simulink model "sampleModel7293_pp_1_1"  (R2018a)
settings: Solver=VariableStepAuto  StartTime=0.0  StopTime=10.0  RelTol=1e-3
undefined symbols (not defined in the file): DiscIntNeverNeededParam
libraries: simulink x367
(part 7 of 12)

== system sampleModel7293_pp_1_1/cfblk175/cfblk17 ==
  cfblk1 : Inport
  cfblk14 : Inport  Port=2
  Action Port : ActionPort  ActionType=else
  cfblk10 : simulink/Continuous/PID Controller (2DOF)  Controller=PID  TimeDomain=Discrete-time  SampleTime=-1  IntegratorMethod=Forward Euler  FilterMethod=Forward Euler  Form=Parallel  UseFilter=on  ControllerParametersSource=internal  P=1  I=1  D=0  N=100  b=1  c=1  InitialConditionSource=internal  InitialConditionForIntegrator=0  InitialConditionForFilter=0  ExternalReset=none  LimitOutput=off  UpperSaturationLimit=inf  LowerSaturationLimit=-inf  LinearizeAsGain=off  AntiWindupMode=none  Kb=1  TrackingMode=off  Kt=1  PParamMin=[]  PParamMax=[]  IParamMin=[]  IParamMax=[]  DParamMin=[]  DParamMax=[]  NParamMin=[]  NParamMax=[]  bParamMin=[]  bParamMax=[]  cParamMin=[]  cParamMax=[]  KbParamMin=[]  KbParamMax=[]  KtParamMin=[]  KtParamMax=[]  POutMin=[]  POutMax=[]  IOutMin=[]  IOutMax=[]  DOutMin=[]  DOutMax=[]  NOutMin=[]  NOutMax=[]  bOutMin=[]  bOutMax=[]  cOutMin=[]  cOutMax=[]  KbOutMin=[]  KbOutMax=[]  KtOutMin=[]  KtOutMax=[]  IntegratorOutMin=[]  IntegratorOutMax=[]  FilterOutMin=[]  FilterOutMax=[]  SumOutMin=[]  SumOutMax=[]  Sum1OutMin=[]  Sum1OutMax=[]  Sum2OutMin=[]  Sum2OutMax=[]  Sum3OutMin=[]  Sum3OutMax=[]  SumI1OutMin=[]  SumI1OutMax=[]  SumI2OutMin=[]  SumI2OutMax=[]  SumI3OutMin=[]  SumI3OutMax=[]  SumDOutMin=[]  SumDOutMax=[]  SaturationOutMin=[]  SaturationOutMax=[]  IntegratorContinuousStateAttributes=''  IntegratorStateMustResolveToSignalObject=off  IntegratorRTWStateStorageClass=Auto  FilterContinuousStateAttributes=''  FilterStateMustResolveToSignalObject=off  FilterRTWStateStorageClass=Auto  DifferentiatorICPrevScaledInput=0  DifferentiatorOutMin=[]  DifferentiatorOutMax=[]  FilterDiffOutCoefMin=[]  FilterDiffOutCoefMax=[]  SumDenOutMin=[]  SumDenOutMax=[]  SumNumOutMin=[]  SumNumOutMax=[]  ReciprocalOutMin=[]  ReciprocalOutMax=[]  DivideOutMin=[]  DivideOutMax=[]  TunerSelectOption=Transfer Function Based (PID Tuner App)
  cfblk11 : simulink/Discrete/Difference  ICPrevInput=0.0  OutMin=[]  OutMax=[]  OutDataTypeStr=double  OutputDataTypeScalingMode=double  OutDataType=fixdt(1, 16)  OutScaling=2^-10  DoSatur=off
  cfblk12 : simulink/Continuous/PID Controller (2DOF)  Controller=PID  TimeDomain=Discrete-time  SampleTime=-1  IntegratorMethod=Forward Euler  FilterMethod=Forward Euler  Form=Parallel  UseFilter=on  ControllerParametersSource=internal  P=1  I=1  D=0  N=100  b=1  c=1  InitialConditionSource=internal  InitialConditionForIntegrator=0  InitialConditionForFilter=0  ExternalReset=none  LimitOutput=off  UpperSaturationLimit=inf  LowerSaturationLimit=-inf  LinearizeAsGain=off  AntiWindupMode=none  Kb=1  TrackingMode=off  Kt=1  PParamMin=[]  PParamMax=[]  IParamMin=[]  IParamMax=[]  DParamMin=[]  DParamMax=[]  NParamMin=[]  NParamMax=[]  bParamMin=[]  bParamMax=[]  cParamMin=[]  cParamMax=[]  KbParamMin=[]  KbParamMax=[]  KtParamMin=[]  KtParamMax=[]  POutMin=[]  POutMax=[]  IOutMin=[]  IOutMax=[]  DOutMin=[]  DOutMax=[]  NOutMin=[]  NOutMax=[]  bOutMin=[]  bOutMax=[]  cOutMin=[]  cOutMax=[]  KbOutMin=[]  KbOutMax=[]  KtOutMin=[]  KtOutMax=[]  IntegratorOutMin=[]  IntegratorOutMax=[]  FilterOutMin=[]  FilterOutMax=[]  SumOutMin=[]  SumOutMax=[]  Sum1OutMin=[]  Sum1OutMax=[]  Sum2OutMin=[]  Sum2OutMax=[]  Sum3OutMin=[]  Sum3OutMax=[]  SumI1OutMin=[]  SumI1OutMax=[]  SumI2OutMin=[]  SumI2OutMax=[]  SumI3OutMin=[]  SumI3OutMax=[]  SumDOutMin=[]  SumDOutMax=[]  SaturationOutMin=[]  SaturationOutMax=[]  IntegratorContinuousStateAttributes=''  IntegratorStateMustResolveToSignalObject=off  IntegratorRTWStateStorageClass=Auto  FilterContinuousStateAttributes=''  FilterStateMustResolveToSignalObject=off  FilterRTWStateStorageClass=Auto  DifferentiatorICPrevScaledInput=0  DifferentiatorOutMin=[]  DifferentiatorOutMax=[]  FilterDiffOutCoefMin=[]  FilterDiffOutCoefMax=[]  SumDenOutMin=[]  SumDenOutMax=[]  SumNumOutMin=[]  SumNumOutMax=[]  ReciprocalOutMin=[]  ReciprocalOutMax=[]  DivideOutMin=[]  DivideOutMax=[]  TunerSelectOption=Transfer Function Based (PID Tuner App)
  cfblk13 : simulink/Discrete/Transfer Fcn Real Zero  ZeroZ=0.75  ICPrevInput=0.0  DoSatur=off
      settings: SourceProductName=Simulink  SourceProductBaseCode=SL
  cfblk16 : Delay
  cfblk3 : Subsystem  TreatAsAtomicUnit=on
  cfblk4 : simulink/Discrete/Tapped Delay  vinit=0.0  samptime=-1  NumDelays=1  DelayOrder=Oldest  includeCurrent=off
  cfblk5 : Subsystem  TreatAsAtomicUnit=on
  cfblk6 : DiscreteIntegrator  SampleTime=-1  OutDataTypeStr=double  ICPrevOutput=DiscIntNeverNeededParam  ICPrevScaledInput=DiscIntNeverNeededParam
  cfblk7 : DiscreteZeroPole  Poles=[0 0.5]  Gain=1  SampleTime=-1
  cfblk8 : Subsystem  TreatAsAtomicUnit=on
  cfblk9 : DiscreteZeroPole  Poles=[0 0.5]  Gain=1  SampleTime=-1
  cyemi_{344..357} (14 alike) : DataTypeConversion  OutDataTypeStr=double
  emi_1488 : Subsystem  TreatAsAtomicUnit=on
  emi_1490 : If  IfExpression=0 <= u1
  emi_1491 : DataTypeConversion  OutDataTypeStr=double
  emi_2063 : Subsystem  TreatAsAtomicUnit=on
  emi_2065 : If  IfExpression=0 <= u1
  emi_2066 : DataTypeConversion  OutDataTypeStr=double
  emi_274 : Subsystem  TreatAsAtomicUnit=on
  emi_276 : If  IfExpression=0 <= u1
  emi_277 : DataTypeConversion  OutDataTypeStr=double
  cfblk2 : Outport
  cfblk15 : Outport  Port=2
  wires:
  cfblk7/1 -> cfblk15/1
  cfblk10/1 -> cfblk2/1
  cfblk12/1 -> cyemi_349/1, cyemi_350/1
  cfblk6/1 -> cyemi_345/1, cyemi_357/1
  cyemi_344/1 -> cfblk10/1
  cfblk13/1 -> cyemi_344/1
  cyemi_345/1 -> cfblk10/2
  cyemi_346/1 -> cfblk11/1
  cfblk9/1 -> cyemi_346/1
  cyemi_347/1 -> cfblk12/1
  cyemi_348/1 -> cfblk12/2
  cfblk14/1 -> cyemi_348/1
  cyemi_349/1 -> cfblk13/1
  cyemi_350/1 -> cfblk16/1
  cyemi_352/1 -> cfblk4/1
  cfblk16/1 -> cyemi_353/1, emi_1491/1, emi_2066/1
  cyemi_354/1 -> cfblk6/1
  cfblk4/1 -> cyemi_354/1, emi_277/1
  cyemi_355/1 -> cfblk7/1
  cfblk11/1 -> cyemi_355/1
  cfblk1/1 -> cyemi_356/1
  cyemi_357/1 -> cfblk9/1
  cyemi_351/1 -> cfblk3/1(emi_272)
  cfblk3/1(emi_273) -> cyemi_352/1
  emi_276/1 -> cfblk3/Action
  emi_276/2 -> emi_274/Action
  emi_277/1 -> emi_276/1
  cyemi_353/1 -> cfblk5/1(emi_1486)
  cfblk5/1(emi_1487) -> cyemi_347/1
  emi_1490/1 -> cfblk5/Action
  emi_1490/2 -> emi_1488/Action
  emi_1491/1 -> emi_1490/1
  cyemi_356/1 -> cfblk8/1(emi_2061)
  cfblk8/1(emi_2062) -> cyemi_351/1
  emi_2065/1 -> cfblk8/Action
  emi_2065/2 -> emi_2063/Action
  emi_2066/1 -> emi_2065/1

== system sampleModel7293_pp_1_1/cfblk175/cfblk5 ==
  emi_193 : Inport
  emi_194 : Inport  Port=2
  Action Port : ActionPort  ActionType=then
  cfblk5 : simulink/Continuous/PID Controller (2DOF)  Controller=PID  TimeDomain=Discrete-time  SampleTime=-1  IntegratorMethod=Forward Euler  FilterMethod=Forward Euler  Form=Parallel  UseFilter=on  ControllerParametersSource=internal  P=1  I=1  D=0  N=100  b=1  c=1  InitialConditionSource=internal  InitialConditionForIntegrator=0  InitialConditionForFilter=0  ExternalReset=none  LimitOutput=off  UpperSaturationLimit=inf  LowerSaturationLimit=-inf  LinearizeAsGain=off  AntiWindupMode=none  Kb=1  TrackingMode=off  Kt=1  PParamMin=[]  PParamMax=[]  IParamMin=[]  IParamMax=[]  DParamMin=[]  DParamMax=[]  NParamMin=[]  NParamMax=[]  bParamMin=[]  bParamMax=[]  cParamMin=[]  cParamMax=[]  KbParamMin=[]  KbParamMax=[]  KtParamMin=[]  KtParamMax=[]  POutMin=[]  POutMax=[]  IOutMin=[]  IOutMax=[]  DOutMin=[]  DOutMax=[]  NOutMin=[]  NOutMax=[]  bOutMin=[]  bOutMax=[]  cOutMin=[]  cOutMax=[]  KbOutMin=[]  KbOutMax=[]  KtOutMin=[]  KtOutMax=[]  IntegratorOutMin=[]  IntegratorOutMax=[]  FilterOutMin=[]  FilterOutMax=[]  SumOutMin=[]  SumOutMax=[]  Sum1OutMin=[]  Sum1OutMax=[]  Sum2OutMin=[]  Sum2OutMax=[]  Sum3OutMin=[]  Sum3OutMax=[]  SumI1OutMin=[]  SumI1OutMax=[]  SumI2OutMin=[]  SumI2OutMax=[]  SumI3OutMin=[]  SumI3OutMax=[]  SumDOutMin=[]  SumDOutMax=[]  SaturationOutMin=[]  SaturationOutMax=[]  IntegratorContinuousStateAttributes=''  IntegratorStateMustResolveToSignalObject=off  IntegratorRTWStateStorageClass=Auto  FilterContinuousStateAttributes=''  FilterStateMustResolveToSignalObject=off  FilterRTWStateStorageClass=Auto  DifferentiatorICPrevScaledInput=0  DifferentiatorOutMin=[]  DifferentiatorOutMax=[]  FilterDiffOutCoefMin=[]  FilterDiffOutCoefMax=[]  SumDenOutMin=[]  SumDenOutMax=[]  SumNumOutMin=[]  SumNumOutMax=[]  ReciprocalOutMin=[]  ReciprocalOutMax=[]  DivideOutMin=[]  DivideOutMax=[]  TunerSelectOption=Transfer Function Based (PID Tuner App)
  emi_195 : Outport
  wires:
  emi_193/1 -> cfblk5/1
  emi_194/1 -> cfblk5/2
  cfblk5/1 -> emi_195/1

== system sampleModel7293_pp_1_1/cfblk175/cfblk6 ==
  emi_502 : Inport
  Action Port : ActionPort  ActionType=then
  cfblk6 : DiscreteFilter
  emi_503 : Outport
  wires:
  emi_502/1 -> cfblk6/1
  cfblk6/1 -> emi_503/1

== system sampleModel7293_pp_1_1/cfblk175/cfblk7 ==
  emi_987 : Inport
  Action Port : ActionPort  ActionType=then
  cfblk7 : DiscreteZeroPole  Poles=[0 0.5]  Gain=1  SampleTime=-1
  emi_988 : Outport
  wires:
  emi_987/1 -> cfblk7/1
  cfblk7/1 -> emi_988/1

== system sampleModel7293_pp_1_1/cfblk175/cfblk8 ==
  emi_315 : Inport
  Action Port : ActionPort  ActionType=then
  cfblk8 : DiscreteFilter
  emi_316 : Outport
  wires:
  emi_315/1 -> cfblk8/1
  cfblk8/1 -> emi_316/1

== system sampleModel7293_pp_1_1/cfblk175/emi_196 ==
  Action Port : ActionPort  ActionType=else
  emi_197 : Assertion

== system sampleModel7293_pp_1_1/cfblk175/emi_317 ==
  Action Port : ActionPort  ActionType=else
  emi_318 : Assertion

== system sampleModel7293_pp_1_1/cfblk175/emi_504 ==
  Action Port : ActionPort  ActionType=else
  emi_505 : Assertion

== system sampleModel7293_pp_1_1/cfblk175/emi_989 ==
  Action Port : ActionPort  ActionType=else
  emi_990 : Assertion

== system sampleModel7293_pp_1_1/cfblk177/cfblk8 ==
  emi_50 : Inport
  Action Port : ActionPort  ActionType=then
  cfblk8 : DiscreteIntegrator  SampleTime=-1  OutDataTypeStr=double  ICPrevOutput=DiscIntNeverNeededParam  ICPrevScaledInput=DiscIntNeverNeededParam
  emi_51 : Outport
  wires:
  emi_50/1 -> cfblk8/1
  cfblk8/1 -> emi_51/1

== system sampleModel7293_pp_1_1/cfblk177/emi_52 ==
  Action Port : ActionPort  ActionType=else
  emi_53 : Assertion

== system sampleModel7293_pp_1_1/cfblk178/cfblk3 ==
  emi_1650 : Inport
  Action Port : ActionPort  ActionType=then
  cfblk3 : simulink/Discrete/Transfer Fcn Real Zero  ZeroZ=0.75  ICPrevInput=0.0  DoSatur=off
      settings: SourceProductName=Simulink  SourceProductBaseCode=SL
  emi_1651 : Outport
  wires:
  emi_1650/1 -> cfblk3/1
  cfblk3/1 -> emi_1651/1

== system sampleModel7293_pp_1_1/cfblk178/cfblk4 ==
  emi_746 : Inport
  Action Port : ActionPort  ActionType=then
  cfblk4 : DiscreteIntegrator  SampleTime=-1  OutDataTypeStr=double  ICPrevOutput=DiscIntNeverNeededParam  ICPrevScaledInput=DiscIntNeverNeededParam
  emi_747 : Outport
  wires:
  emi_746/1 -> cfblk4/1
  cfblk4/1 -> emi_747/1

== system sampleModel7293_pp_1_1/cfblk178/cfblk9 ==
  emi_2019 : Inport
  Action Port : ActionPort  ActionType=then
  cfblk9 : DiscreteZeroPole  Poles=[0 0.5]  Gain=1  SampleTime=-1
  emi_2020 : Outport
  wires:
  emi_2019/1 -> cfblk9/1
  cfblk9/1 -> emi_2020/1

== system sampleModel7293_pp_1_1/cfblk178/emi_1652 ==
  Action Port : ActionPort  ActionType=else
  emi_1653 : Assertion

== system sampleModel7293_pp_1_1/cfblk178/emi_2021 ==
  Action Port : ActionPort  ActionType=else
  emi_2022 : Assertion

== system sampleModel7293_pp_1_1/cfblk178/emi_748 ==
  Action Port : ActionPort  ActionType=else
  emi_749 : Assertion

== system sampleModel7293_pp_1_1/cfblk179/cfblk16 ==
  emi_1287 : Inport
  Action Port : ActionPort  ActionType=then
  cfblk16 : Delay
  emi_1288 : Outport
  wires:
  emi_1287/1 -> cfblk16/1
  cfblk16/1 -> emi_1288/1

== system sampleModel7293_pp_1_1/cfblk179/cfblk7 ==
  emi_57 : Inport
  Action Port : ActionPort  ActionType=then
  cfblk7 : simulink/Discrete/Transfer Fcn Lead or Lag  PoleZ=0.95  ZeroZ=0.75  ICPrevOutput=0.0  ICPrevInput=0.0  DoSatur=off
      settings: SourceProductName=Simulink  SourceProductBaseCode=SL
  emi_58 : Outport
  wires:
  emi_57/1 -> cfblk7/1
  cfblk7/1 -> emi_58/1

== system sampleModel7293_pp_1_1/cfblk179/cfblk8 ==
  emi_1600 : Inport
  Action Port : ActionPort  ActionType=then
  cfblk8 : simulink/Discrete/Transfer Fcn Real Zero  ZeroZ=0.75  ICPrevInput=0.0  DoSatur=off
      settings: SourceProductName=Simulink  SourceProductBaseCode=SL
  emi_1601 : Outport
  wires:
  emi_1600/1 -> cfblk8/1
  cfblk8/1 -> emi_1601/1

== system sampleModel7293_pp_1_1/cfblk179/emi_1289 ==
  Action Port : ActionPort  ActionType=else
  emi_1290 : Assertion

== system sampleModel7293_pp_1_1/cfblk179/emi_1602 ==
  Action Port : ActionPort  ActionType=else
  emi_1603 : Assertion

== system sampleModel7293_pp_1_1/cfblk179/emi_59 ==
  Action Port : ActionPort  ActionType=else
  emi_60 : Assertion

== system sampleModel7293_pp_1_1/cfblk180/cfblk17 ==
  cfblk1 : Inport
  Action Port : ActionPort  ActionType=then
  cfblk10 : Delay
  cfblk3 : Subsystem  TreatAsAtomicUnit=on
  cfblk4 : Delay  ShowEnablePort=on
      settings: InputPortMap=u0,e6
  cfblk5 : Subsystem  TreatAsAtomicUnit=on
  cfblk6 : DiscreteTransferFcn
  cfblk7 : Subsystem  TreatAsAtomicUnit=on
  cfblk8 : Subsystem  TreatAsAtomicUnit=on
  cfblk9 : Subsystem  TreatAsAtomicUnit=on
  cyemi_{429..439} (11 alike) : DataTypeConversion  OutDataTypeStr=double
  emi_110 : Subsystem  TreatAsAtomicUnit=on
  emi_{112,356,822,1505,1931} (5 alike) : If  IfExpression=Inf <= u1
  emi_{113,357,823,1506,1932} (5 alike) : DataTypeConversion  OutDataTypeStr=double
  emi_1503 : Subsystem  TreatAsAtomicUnit=on
  emi_1929 : Subsystem  TreatAsAtomicUnit=on
  emi_354 : Subsystem  TreatAsAtomicUnit=on
  emi_820 : Subsystem  TreatAsAtomicUnit=on
  cfblk2 : Outport
  wires:
  cfblk1/1 -> cyemi_434/1, cyemi_436/1, cyemi_437/1
  cyemi_429/1 -> cfblk10/1
  cfblk6/1 -> cyemi_431/1, emi_823/1
  cyemi_432/1 -> cfblk4/1
  cyemi_433/1 -> cfblk4/2
  cfblk10/1 -> cyemi_433/1, emi_1506/1, emi_1932/1
  cyemi_435/1 -> cfblk6/1
  cfblk4/1 -> cyemi_439/1, emi_357/1
  cyemi_439/1 -> cfblk9/1(emi_108)
  cfblk9/1(emi_109) -> cyemi_438/1, cyemi_430/1
  emi_112/1 -> cfblk9/Action
  emi_112/2 -> emi_110/Action
  emi_113/1 -> emi_112/1
  cyemi_438/1 -> cfblk8/1(emi_352)
  cfblk8/1(emi_353) -> cyemi_429/1
  emi_356/1 -> cfblk8/Action
  emi_356/2 -> emi_354/Action
  emi_357/1 -> emi_356/1
  cyemi_430/1 -> cfblk3/1(emi_817)
  cyemi_431/1 -> cfblk3/2(emi_818)
  cfblk3/1(emi_819) -> cfblk2/1
  emi_822/1 -> cfblk3/Action
  emi_822/2 -> emi_820/Action
  emi_823/1 -> emi_822/1
  cyemi_436/1 -> cfblk7/1(emi_1500)
  cyemi_437/1 -> cfblk7/2(emi_1501)
  cfblk7/1(emi_1502) -> cyemi_435/1
  emi_1505/1 -> cfblk7/Action
  emi_1505/2 -> emi_1503/Action
  emi_1506/1 -> emi_1505/1
  cyemi_434/1 -> cfblk5/1(emi_1927)
  cfblk5/1(emi_1928) -> emi_113/1, cyemi_432/1
  emi_1931/1 -> cfblk5/Action
  emi_1931/2 -> emi_1929/Action
  emi_1932/1 -> emi_1931/1

== system sampleModel7293_pp_1_1/cfblk180/cfblk18 ==
  cfblk1 : Inport
  Action Port : ActionPort  ActionType=else
  cfblk10 : Subsystem  TreatAsAtomicUnit=on
  cfblk11 : simulink/Continuous/PID Controller  Controller=PID  TimeDomain=Discrete-time  SampleTime=-1  IntegratorMethod=Forward Euler  FilterMethod=Forward Euler  Form=Parallel  UseFilter=on  ControllerParametersSource=internal  P=1  I=1  D=0  N=100  InitialConditionSource=internal  InitialConditionForIntegrator=0  InitialConditionForFilter=0  ExternalReset=none  LimitOutput=off  UpperSaturationLimit=inf  LowerSaturationLimit=-inf  LinearizeAsGain=off  AntiWindupMode=none  Kb=1  TrackingMode=off  Kt=1  PParamMin=[]  PParamMax=[]  IParamMin=[]  IParamMax=[]  DParamMin=[]  DParamMax=[]  NParamMin=[]  NParamMax=[]  KbParamMin=[]  KbParamMax=[]  KtParamMin=[]  KtParamMax=[]  POutMin=[]  POutMax=[]  IOutMin=[]  IOutMax=[]  DOutMin=[]  DOutMax=[]  NOutMin=[]  NOutMax=[]  KbOutMin=[]  KbOutMax=[]  KtOutMin=[]  KtOutMax=[]  IntegratorOutMin=[]  IntegratorOutMax=[]  FilterOutMin=[]  FilterOutMax=[]  SumOutMin=[]  SumOutMax=[]  SumI1OutMin=[]  SumI1OutMax=[]  SumI2OutMin=[]  SumI2OutMax=[]  SumI3OutMin=[]  SumI3OutMax=[]  SumDOutMin=[]  SumDOutMax=[]  SaturationOutMin=[]  SaturationOutMax=[]  IntegratorContinuousStateAttributes=''  IntegratorStateMustResolveToSignalObject=off  IntegratorRTWStateStorageClass=Auto  FilterContinuousStateAttributes=''  FilterStateMustResolveToSignalObject=off  FilterRTWStateStorageClass=Auto  DifferentiatorICPrevScaledInput=0  DifferentiatorOutMin=[]  DifferentiatorOutMax=[]  FilterDiffOutCoefMin=[]  FilterDiffOutCoefMax=[]  SumDenOutMin=[]  SumDenOutMax=[]  SumNumOutMin=[]  SumNumOutMax=[]  ReciprocalOutMin=[]  ReciprocalOutMax=[]  DivideOutMin=[]  DivideOutMax=[]  TunerSelectOption=Transfer Function Based (PID Tuner App)
  cfblk14 : Delay
  cfblk15 : Delay
  cfblk3 : simulink/Discrete/Difference  ICPrevInput=0.0  OutMin=[]  OutMax=[]  OutDataTypeStr=double  OutputDataTypeScalingMode=double  OutDataType=fixdt(1, 16)  OutScaling=2^-10  DoSatur=off
  cfblk4 : simulink/Continuous/PID Controller  Controller=PID  TimeDomain=Discrete-time  SampleTime=-1  IntegratorMethod=Forward Euler  FilterMethod=Forward Euler  Form=Parallel  UseFilter=on  ControllerParametersSource=internal  P=1  I=1  D=0  N=100  InitialConditionSource=internal  InitialConditionForIntegrator=0  InitialConditionForFilter=0  ExternalReset=none  LimitOutput=off  UpperSaturationLimit=inf  LowerSaturationLimit=-inf  LinearizeAsGain=off  AntiWindupMode=none  Kb=1  TrackingMode=off  Kt=1  PParamMin=[]  PParamMax=[]  IParamMin=[]  IParamMax=[]  DParamMin=[]  DParamMax=[]  NParamMin=[]  NParamMax=[]  KbParamMin=[]  KbParamMax=[]  KtParamMin=[]  KtParamMax=[]  POutMin=[]  POutMax=[]  IOutMin=[]  IOutMax=[]  DOutMin=[]  DOutMax=[]  NOutMin=[]  NOutMax=[]  KbOutMin=[]  KbOutMax=[]  KtOutMin=[]  KtOutMax=[]  IntegratorOutMin=[]  IntegratorOutMax=[]  FilterOutMin=[]  FilterOutMax=[]  SumOutMin=[]  SumOutMax=[]  SumI1OutMin=[]  SumI1OutMax=[]  SumI2OutMin=[]  SumI2OutMax=[]  SumI3OutMin=[]  SumI3OutMax=[]  SumDOutMin=[]  SumDOutMax=[]  SaturationOutMin=[]  SaturationOutMax=[]  IntegratorContinuousStateAttributes=''  IntegratorStateMustResolveToSignalObject=off  IntegratorRTWStateStorageClass=Auto  FilterContinuousStateAttributes=''  FilterStateMustResolveToSignalObject=off  FilterRTWStateStorageClass=Auto  DifferentiatorICPrevScaledInput=0  DifferentiatorOutMin=[]  DifferentiatorOutMax=[]  FilterDiffOutCoefMin=[]  FilterDiffOutCoefMax=[]  SumDenOutMin=[]  SumDenOutMax=[]  SumNumOutMin=[]  SumNumOutMax=[]  ReciprocalOutMin=[]  ReciprocalOutMax=[]  DivideOutMin=[]  DivideOutMax=[]  TunerSelectOption=Transfer Function Based (PID Tuner App)
  cfblk5 : Subsystem  TreatAsAtomicUnit=on
  cfblk6 : Delay
  cfblk7 : Subsystem  TreatAsAtomicUnit=on
  cfblk8 : Delay  DelayLengthSource=Input port
      settings: InputPortMap=u0,p1
  cfblk9 : Delay  ShowEnablePort=on
      settings: InputPortMap=u0,e6
  cyemi_{441..454} (14 alike) : DataTypeConversion  OutDataTypeStr=double
  emi_2085 : Subsystem  TreatAsAtomicUnit=on
  emi_2087 : If  IfExpression=Inf <= u1
  emi_2088 : DataTypeConversion  OutDataTypeStr=double
  emi_2107 : Subsystem  TreatAsAtomicUnit=on
  emi_2109 : If  IfExpression=Inf <= u1
  emi_2110 : DataTypeConversion  OutDataTypeStr=double
  emi_238 : Subsystem  TreatAsAtomicUnit=on
  emi_240 : If  IfExpression=Inf <= u1
  emi_241 : DataTypeConversion  OutDataTypeStr=double
  cfblk2 : Outport
  cfblk12 : Outport  Port=2
  cfblk13 : Outport  Port=3
  wires:
  cfblk4/1 -> cyemi_449/1, cyemi_454/1
  cfblk8/1 -> cfblk2/1, cyemi_446/1
  cfblk3/1 -> cyemi_441/1, cyemi_450/1
  cfblk6/1 -> cyemi_445/1, cyemi_453/1, emi_241/1, emi_2088/1
  cyemi_442/1 -> cfblk11/1
  cyemi_443/1 -> cfblk14/1
  cfblk11/1 -> cyemi_443/1
  cyemi_444/1 -> cfblk15/1
  cfblk9/1 -> cyemi_444/1
  cyemi_445/1 -> cfblk3/1
  cyemi_446/1 -> cfblk4/1
  cfblk15/1 -> cyemi_447/1, emi_2110/1
  cfblk1/1 -> cyemi_448/1
  cyemi_449/1 -> cfblk6/1
  cyemi_451/1 -> cfblk8/1
  cyemi_452/1 -> cfblk8/2
  cfblk14/1 -> cyemi_452/1
  cyemi_453/1 -> cfblk9/1
  cyemi_454/1 -> cfblk9/2
  cyemi_450/1 -> cfblk7/1(emi_236)
  cfblk7/1(emi_237) -> cfblk12/1
  emi_240/1 -> cfblk7/Action
  emi_240/2 -> emi_238/Action
  emi_241/1 -> emi_240/1
  cyemi_447/1 -> cfblk5/1(emi_2082)
  cyemi_448/1 -> cfblk5/2(emi_2083)
  cfblk5/1(emi_2084) -> cyemi_451/1, cfblk13/1
  emi_2087/1 -> cfblk5/Action
  emi_2087/2 -> emi_2085/Action
  emi_2088/1 -> emi_2087/1
  cyemi_441/1 -> cfblk10/1(emi_2105)
  cfblk10/1(emi_2106) -> cyemi_442/1
  emi_2109/1 -> cfblk10/Action
  emi_2109/2 -> emi_2107/Action
  emi_2110/1 -> emi_2109/1

== system sampleModel7293_pp_1_1/cfblk180/cfblk4 ==
  emi_1998 : Inport
  Action Port : ActionPort  ActionType=then
  cfblk4 : Delay
  emi_1999 : Outport
  wires:
  emi_1998/1 -> cfblk4/1
  cfblk4/1 -> emi_1999/1

== system sampleModel7293_pp_1_1/cfblk180/cfblk9 ==
  emi_2133 : Inport
  Action Port : ActionPort  ActionType=then
  cfblk9 : DiscreteZeroPole  Poles=[0 0.5]  Gain=1  SampleTime=-1
  emi_2134 : Outport
  wires:
  emi_2133/1 -> cfblk9/1
  cfblk9/1 -> emi_2134/1

== system sampleModel7293_pp_1_1/cfblk180/emi_2000 ==
  Action Port : ActionPort  ActionType=else
  emi_2001 : Assertion

== system sampleModel7293_pp_1_1/cfblk180/emi_2135 ==
  Action Port : ActionPort  ActionType=else
  emi_2136 : Assertion

== system sampleModel7293_pp_1_1/cfblk181/cfblk10 ==
  emi_79 : Inport
  Action Port : ActionPort  ActionType=then
  cfblk10 : Delay
  emi_80 : Outport
  wires:
  emi_79/1 -> cfblk10/1
  cfblk10/1 -> emi_80/1

== system sampleModel7293_pp_1_1/cfblk181/emi_81 ==
  Action Port : ActionPort  ActionType=else
  emi_82 : Assertion

== system sampleModel7293_pp_1_1/cfblk182/cfblk12 ==
  cfblk1 : Inport
  cfblk13 : Inport  Port=2
  cfblk14 : Inport  Port=3
  Action Port : ActionPort  ActionType=then
  cfblk10 : simulink/Discrete/Transfer Fcn Real Zero  ZeroZ=0.75  ICPrevInput=0.0  DoSatur=off
      settings: SourceProductName=Simulink  SourceProductBaseCode=SL
  cfblk11 : simulink/Discrete/Transfer Fcn First Order  PoleZ=0.95  ICPrevOutput=0.0  DoSatur=off
      settings: SourceProductName=Simulink
  cfblk12 : simulink/Discrete/Tapped Delay  vinit=0.0  samptime=-1  NumDelays=1  DelayOrder=Oldest  includeCurrent=off
  cfblk3 : Subsystem  TreatAsAtomicUnit=on
  cfblk4 : DiscreteFir
  cfblk5 : DiscreteFilter
  cfblk6 : DiscreteFir
  cfblk7 : Subsystem  TreatAsAtomicUnit=on
  cfblk8 : Delay  ShowEnablePort=on
      settings: InputPortMap=u0,e6
  cfblk9 : simulink/Continuous/PID Controller  Controller=PID  TimeDomain=Discrete-time  SampleTime=-1  IntegratorMethod=Forward Euler  FilterMethod=Forward Euler  Form=Parallel  UseFilter=on  ControllerParametersSource=internal  P=1  I=1  D=0  N=100  InitialConditionSource=internal  InitialConditionForIntegrator=0  InitialConditionForFilter=0  ExternalReset=none  LimitOutput=off  UpperSaturationLimit=inf  LowerSaturationLimit=-inf  LinearizeAsGain=off  AntiWindupMode=none  Kb=1  TrackingMode=off  Kt=1  PParamMin=[]  PParamMax=[]  IParamMin=[]  IParamMax=[]  DParamMin=[]  DParamMax=[]  NParamMin=[]  NParamMax=[]  KbParamMin=[]  KbParamMax=[]  KtParamMin=[]  KtParamMax=[]  POutMin=[]  POutMax=[]  IOutMin=[]  IOutMax=[]  DOutMin=[]  DOutMax=[]  NOutMin=[]  NOutMax=[]  KbOutMin=[]  KbOutMax=[]  KtOutMin=[]  KtOutMax=[]  IntegratorOutMin=[]  IntegratorOutMax=[]  FilterOutMin=[]  FilterOutMax=[]  SumOutMin=[]  SumOutMax=[]  SumI1OutMin=[]  SumI1OutMax=[]  SumI2OutMin=[]  SumI2OutMax=[]  SumI3OutMin=[]  SumI3OutMax=[]  SumDOutMin=[]  SumDOutMax=[]  SaturationOutMin=[]  SaturationOutMax=[]  IntegratorContinuousStateAttributes=''  IntegratorStateMustResolveToSignalObject=off  IntegratorRTWStateStorageClass=Auto  FilterContinuousStateAttributes=''  FilterStateMustResolveToSignalObject=off  FilterRTWStateStorageClass=Auto  DifferentiatorICPrevScaledInput=0  DifferentiatorOutMin=[]  DifferentiatorOutMax=[]  FilterDiffOutCoefMin=[]  FilterDiffOutCoefMax=[]  SumDenOutMin=[]  SumDenOutMax=[]  SumNumOutMin=[]  SumNumOutMax=[]  ReciprocalOutMin=[]  ReciprocalOutMax=[]  DivideOutMin=[]  DivideOutMax=[]  TunerSelectOption=Transfer Function Based (PID Tuner App)
  cyemi_{480..490} (11 alike) : DataTypeConversion  OutDataTypeStr=double
  emi_103 : Subsystem  TreatAsAtomicUnit=on
  emi_105 : If  IfExpression=Inf <= u1
  emi_106 : DataTypeConversion  OutDataTypeStr=double
  emi_982 : Subsystem  TreatAsAtomicUnit=on
  emi_984 : If  IfExpression=Inf <= u1
  emi_985 : DataTypeConversion  OutDataTypeStr=double
  cfblk2 : Outport
  wires:
  cfblk11/1 -> cfblk2/1
  cyemi_480/1 -> cfblk10/1
  cyemi_481/1 -> cfblk11/1
  cfblk14/1 -> cyemi_481/1
  cyemi_482/1 -> cfblk12/1
  cfblk1/1 -> cyemi_482/1
  cfblk13/1 -> cyemi_483/1
  cyemi_484/1 -> cfblk4/1
  cfblk9/1 -> cyemi_484/1
  cyemi_485/1 -> cfblk5/1
  cfblk4/1 -> cyemi_485/1, emi_106/1
  cyemi_486/1 -> cfblk6/1
  cfblk8/1 -> cyemi_486/1
  cyemi_488/1 -> cfblk8/1
  cfblk12/1 -> cyemi_488/1, emi_985/1
  cyemi_489/1 -> cfblk8/2
  cfblk5/1 -> cyemi_489/1
  cyemi_490/1 -> cfblk9/1
  cfblk10/1 -> cyemi_490/1
  cyemi_487/1 -> cfblk7/1(emi_101)
  cfblk7/1(emi_102) -> cyemi_480/1
  emi_105/1 -> cfblk7/Action
  emi_105/2 -> emi_103/Action
  emi_106/1 -> emi_105/1
  cyemi_483/1 -> cfblk3/1(emi_980)
  cfblk3/1(emi_981) -> cyemi_487/1
  emi_984/1 -> cfblk3/Action
  emi_984/2 -> emi_982/Action
  emi_985/1 -> emi_984/1

== system sampleModel7293_pp_1_1/cfblk182/cfblk13 ==
  cfblk1 : Inport
  cfblk9 : Inport  Port=2
  cfblk10 : Inport  Port=3
  Action Port : ActionPort  ActionType=else
  cfblk11 : Subsystem  TreatAsAtomicUnit=on
  cfblk3 : Subsystem  TreatAsAtomicUnit=on
  cfblk4 : DiscreteIntegrator  SampleTime=-1  OutDataTypeStr=double  ICPrevOutput=DiscIntNeverNeededParam  ICPrevScaledInput=DiscIntNeverNeededParam
  cfblk5 : DiscreteZeroPole  Poles=[0 0.5]  Gain=1  SampleTime=-1
  cfblk6 : DiscreteIntegrator  SampleTime=-1  OutDataTypeStr=double  ICPrevOutput=DiscIntNeverNeededParam  ICPrevScaledInput=DiscIntNeverNeededParam
  cfblk7 : DiscreteZeroPole  Poles=[0 0.5]  Gain=1  SampleTime=-1
  cfblk8 : simulink/Continuous/PID Controller (2DOF)  Controller=PID  TimeDomain=Discrete-time  SampleTime=-1  IntegratorMethod=Forward Euler  FilterMethod=Forward Euler  Form=Parallel  UseFilter=on  ControllerParametersSource=internal  P=1  I=1  D=0  N=100  b=1  c=1  InitialConditionSource=internal  InitialConditionForIntegrator=0  InitialConditionForFilter=0  ExternalReset=none  LimitOutput=off  UpperSaturationLimit=inf  LowerSaturationLimit=-inf  LinearizeAsGain=off  AntiWindupMode=none  Kb=1  TrackingMode=off  Kt=1  PParamMin=[]  PParamMax=[]  IParamMin=[]  IParamMax=[]  DParamMin=[]  DParamMax=[]  NParamMin=[]  NParamMax=[]  bParamMin=[]  bParamMax=[]  cParamMin=[]  cParamMax=[]  KbParamMin=[]  KbParamMax=[]  KtParamMin=[]  KtParamMax=[]  POutMin=[]  POutMax=[]  IOutMin=[]  IOutMax=[]  DOutMin=[]  DOutMax=[]  NOutMin=[]  NOutMax=[]  bOutMin=[]  bOutMax=[]  cOutMin=[]  cOutMax=[]  KbOutMin=[]  KbOutMax=[]  KtOutMin=[]  KtOutMax=[]  IntegratorOutMin=[]  IntegratorOutMax=[]  FilterOutMin=[]  FilterOutMax=[]  SumOutMin=[]  SumOutMax=[]  Sum1OutMin=[]  Sum1OutMax=[]  Sum2OutMin=[]  Sum2OutMax=[]  Sum3OutMin=[]  Sum3OutMax=[]  SumI1OutMin=[]  SumI1OutMax=[]  SumI2OutMin=[]  SumI2OutMax=[]  SumI3OutMin=[]  SumI3OutMax=[]  SumDOutMin=[]  SumDOutMax=[]  SaturationOutMin=[]  SaturationOutMax=[]  IntegratorContinuousStateAttributes=''  IntegratorStateMustResolveToSignalObject=off  IntegratorRTWStateStorageClass=Auto  FilterContinuousStateAttributes=''  FilterStateMustResolveToSignalObject=off  FilterRTWStateStorageClass=Auto  DifferentiatorICPrevScaledInput=0  DifferentiatorOutMin=[]  DifferentiatorOutMax=[]  FilterDiffOutCoefMin=[]  FilterDiffOutCoefMax=[]  SumDenOutMin=[]  SumDenOutMax=[]  SumNumOutMin=[]  SumNumOutMax=[]  ReciprocalOutMin=[]  ReciprocalOutMax=[]  DivideOutMin=[]  DivideOutMax=[]  TunerSelectOption=Transfer Function Based (PID Tuner App)
  cyemi_{494..501} (8 alike) : DataTypeConversion  OutDataTypeStr=double
  emi_1466 : Subsystem  TreatAsAtomicUnit=on
  emi_1468 : If  IfExpression=Inf <= u1
  emi_1469 : DataTypeConversion  OutDataTypeStr=double
  emi_1674 : Subsystem  TreatAsAtomicUnit=on
  emi_1676 : If  IfExpression=Inf <= u1
  emi_1677 : DataTypeConversion  OutDataTypeStr=double
  cfblk2 : Outport
  wires:
  cfblk8/1 -> cyemi_494/1
  cfblk5/1 -> cyemi_495/1, emi_1469/1, emi_1677/1
  cyemi_496/1 -> cfblk4/1
  cfblk1/1 -> cyemi_496/1
  cyemi_497/1 -> cfblk5/1
  cfblk6/1 -> cyemi_497/1
  cyemi_498/1 -> cfblk6/1
  cfblk9/1 -> cyemi_498/1
  cyemi_499/1 -> cfblk7/1
  cyemi_500/1 -> cfblk8/1
  cfblk7/1 -> cyemi_500/1
  cyemi_501/1 -> cfblk8/2
  cfblk10/1 -> cyemi_501/1
  cyemi_494/1 -> cfblk11/1(emi_1464)
  cfblk11/1(emi_1465) -> cyemi_499/1
  emi_1468/1 -> cfblk11/Action
  emi_1468/2 -> emi_1466/Action
  emi_1469/1 -> emi_1468/1
  cyemi_495/1 -> cfblk3/1(emi_1672)
  cfblk3/1(emi_1673) -> cfblk2/1
  emi_1676/1 -> cfblk3/Action
  emi_1676/2 -> emi_1674/Action
  emi_1677/1 -> emi_1676/1

== system sampleModel7293_pp_1_1/cfblk182/cfblk15 ==
  emi_1721 : Inport
  Action Port : ActionPort  ActionType=then
  cfblk15 : Delay
  emi_1722 : Outport
  wires:
  emi_1721/1 -> cfblk15/1
  cfblk15/1 -> emi_1722/1

== system sampleModel7293_pp_1_1/cfblk182/cfblk16 ==
  emi_1422 : Inport
  Action Port : ActionPort  ActionType=then
  cfblk16 : Delay
  emi_1423 : Outport
  wires:
  emi_1422/1 -> cfblk16/1
  cfblk16/1 -> emi_1423/1

== system sampleModel7293_pp_1_1/cfblk182/cfblk3 ==
  emi_603 : Inport
  Action Port : ActionPort  ActionType=then
  cfblk3 : simulink/Discrete/Transfer Fcn Lead or Lag  PoleZ=0.95  ZeroZ=0.75  ICPrevOutput=0.0  ICPrevInput=0.0  DoSatur=off
      settings: SourceProductName=Simulink  SourceProductBaseCode=SL
  emi_604 : Outport
  wires:
  emi_603/1 -> cfblk3/1
  cfblk3/1 -> emi_604/1

== system sampleModel7293_pp_1_1/cfblk182/cfblk6 ==
  emi_896 : Inport
  Action Port : ActionPort  ActionType=then
  cfblk6 : UnitDelay  SampleTime=-1
  emi_897 : Outport
  wires:
  emi_896/1 -> cfblk6/1
  cfblk6/1 -> emi_897/1

== system sampleModel7293_pp_1_1/cfblk182/cfblk9 ==
  emi_1771 : Inport
  emi_1772 : Inport  Port=2
  Action Port : ActionPort  ActionType=then
  cfblk9 : Delay  DelayLengthSource=Input port
      settings: InputPortMap=u0,p1
  emi_1773 : Outport
  wires:
  emi_1771/1 -> cfblk9/1
  emi_1772/1 -> cfblk9/2
  cfblk9/1 -> emi_1773/1

== system sampleModel7293_pp_1_1/cfblk182/emi_1424 ==
  Action Port : ActionPort  ActionType=else
  emi_1425 : Assertion

== system sampleModel7293_pp_1_1/cfblk182/emi_1723 ==
  Action Port : ActionPort  ActionType=else
  emi_1724 : Assertion

== system sampleModel7293_pp_1_1/cfblk182/emi_1774 ==
  Action Port : ActionPort  ActionType=else
  emi_1775 : Assertion

== system sampleModel7293_pp_1_1/cfblk182/emi_605 ==
  Action Port : ActionPort  ActionType=else
  emi_606 : Assertion

== system sampleModel7293_pp_1_1/cfblk182/emi_898 ==
  Action Port : ActionPort  ActionType=else
  emi_899 : Assertion

== system sampleModel7293_pp_1_1/cfblk183/cfblk15 ==
  emi_1850 : Inport
  Action Port : ActionPort  ActionType=then
  cfblk15 : Delay
  emi_1851 : Outport
  wires:
  emi_1850/1 -> cfblk15/1
  cfblk15/1 -> emi_1851/1

== system sampleModel7293_pp_1_1/cfblk183/cfblk3 ==
  emi_1400 : Inport
  emi_1401 : Inport  Port=2
  Action Port : ActionPort  ActionType=then
  cfblk3 : Delay  ShowEnablePort=on
      settings: InputPortMap=u0,e6
  emi_1402 : Outport
  wires:
  emi_1400/1 -> cfblk3/1
  emi_1401/1 -> cfblk3/2
  cfblk3/1 -> emi_1402/1

== system sampleModel7293_pp_1_1/cfblk183/cfblk4 ==
  emi_394 : Inport
  Action Port : ActionPort  ActionType=then
  cfblk4 : DiscreteFilter
  emi_395 : Outport
  wires:
  emi_394/1 -> cfblk4/1
  cfblk4/1 -> emi_395/1

== system sampleModel7293_pp_1_1/cfblk183/cfblk5 ==
  emi_1962 : Inport
  Action Port : ActionPort  ActionType=then
  cfblk5 : DiscreteStateSpace  SampleTime=-1
  emi_1963 : Outport
  wires:
  emi_1962/1 -> cfblk5/1
  cfblk5/1 -> emi_1963/1

== system sampleModel7293_pp_1_1/cfblk183/emi_1403 ==
  Action Port : ActionPort  ActionType=else
  emi_1404 : Assertion

== system sampleModel7293_pp_1_1/cfblk183/emi_1852 ==
  Action Port : ActionPort  ActionType=else
  emi_1853 : Assertion

== system sampleModel7293_pp_1_1/cfblk183/emi_1964 ==
  Action Port : ActionPort  ActionType=else
  emi_1965 : Assertion

== system sampleModel7293_pp_1_1/cfblk183/emi_396 ==
  Action Port : ActionPort  ActionType=else
  emi_397 : Assertion

== system sampleModel7293_pp_1_1/cfblk184/cfblk12 ==
  emi_853 : Inport
  emi_854 : Inport  Port=2
  Action Port : ActionPort  ActionType=then
  cfblk12 : simulink/Continuous/PID Controller (2DOF)  Controller=PID  TimeDomain=Discrete-time  SampleTime=-1  IntegratorMethod=Forward Euler  FilterMethod=Forward Euler  Form=Parallel  UseFilter=on  ControllerParametersSource=internal  P=1  I=1  D=0  N=100  b=1  c=1  InitialConditionSource=internal  InitialConditionForIntegrator=0  InitialConditionForFilter=0  ExternalReset=none  LimitOutput=off  UpperSaturationLimit=inf  LowerSaturationLimit=-inf  LinearizeAsGain=off  AntiWindupMode=none  Kb=1  TrackingMode=off  Kt=1  PParamMin=[]  PParamMax=[]  IParamMin=[]  IParamMax=[]  DParamMin=[]  DParamMax=[]  NParamMin=[]  NParamMax=[]  bParamMin=[]  bParamMax=[]  cParamMin=[]  cParamMax=[]  KbParamMin=[]  KbParamMax=[]  KtParamMin=[]  KtParamMax=[]  POutMin=[]  POutMax=[]  IOutMin=[]  IOutMax=[]  DOutMin=[]  DOutMax=[]  NOutMin=[]  NOutMax=[]  bOutMin=[]  bOutMax=[]  cOutMin=[]  cOutMax=[]  KbOutMin=[]  KbOutMax=[]  KtOutMin=[]  KtOutMax=[]  IntegratorOutMin=[]  IntegratorOutMax=[]  FilterOutMin=[]  FilterOutMax=[]  SumOutMin=[]  SumOutMax=[]  Sum1OutMin=[]  Sum1OutMax=[]  Sum2OutMin=[]  Sum2OutMax=[]  Sum3OutMin=[]  Sum3OutMax=[]  SumI1OutMin=[]  SumI1OutMax=[]  SumI2OutMin=[]  SumI2OutMax=[]  SumI3OutMin=[]  SumI3OutMax=[]  SumDOutMin=[]  SumDOutMax=[]  SaturationOutMin=[]  SaturationOutMax=[]  IntegratorContinuousStateAttributes=''  IntegratorStateMustResolveToSignalObject=off  IntegratorRTWStateStorageClass=Auto  FilterContinuousStateAttributes=''  FilterStateMustResolveToSignalObject=off  FilterRTWStateStorageClass=Auto  DifferentiatorICPrevScaledInput=0  DifferentiatorOutMin=[]  DifferentiatorOutMax=[]  FilterDiffOutCoefMin=[]  FilterDiffOutCoefMax=[]  SumDenOutMin=[]  SumDenOutMax=[]  SumNumOutMin=[]  SumNumOutMax=[]  ReciprocalOutMin=[]  ReciprocalOutMax=[]  DivideOutMin=[]  DivideOutMax=[]  TunerSelectOption=Transfer Function Based (PID Tuner App)
  emi_855 : Outport
  wires:
  emi_853/1 -> cfblk12/1
  emi_854/1 -> cfblk12/2
  cfblk12/1 -> emi_855/1

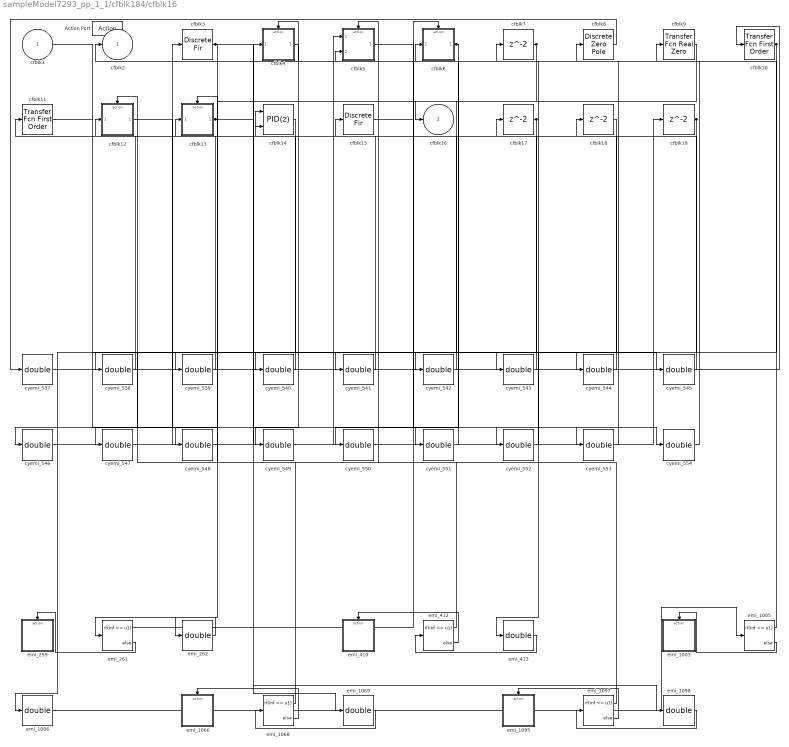
== system sampleModel7293_pp_1_1/cfblk184/cfblk16 ==
  cfblk1 : Inport
  Action Port : ActionPort  ActionType=then
  cfblk10 : simulink/Discrete/Transfer Fcn First Order  PoleZ=0.95  ICPrevOutput=0.0  DoSatur=off
      settings: SourceProductName=Simulink
  cfblk11 : simulink/Discrete/Transfer Fcn First Order  PoleZ=0.95  ICPrevOutput=0.0  DoSatur=off
      settings: SourceProductName=Simulink
  cfblk12 : Subsystem  TreatAsAtomicUnit=on
  cfblk13 : Subsystem  TreatAsAtomicUnit=on
  cfblk14 : simulink/Continuous/PID Controller (2DOF)  Controller=PID  TimeDomain=Discrete-time  SampleTime=-1  IntegratorMethod=Forward Euler  FilterMethod=Forward Euler  Form=Parallel  UseFilter=on  ControllerParametersSource=internal  P=1  I=1  D=0  N=100  b=1  c=1  InitialConditionSource=internal  InitialConditionForIntegrator=0  InitialConditionForFilter=0  ExternalReset=none  LimitOutput=off  UpperSaturationLimit=inf  LowerSaturationLimit=-inf  LinearizeAsGain=off  AntiWindupMode=none  Kb=1  TrackingMode=off  Kt=1  PParamMin=[]  PParamMax=[]  IParamMin=[]  IParamMax=[]  DParamMin=[]  DParamMax=[]  NParamMin=[]  NParamMax=[]  bParamMin=[]  bParamMax=[]  cParamMin=[]  cParamMax=[]  KbParamMin=[]  KbParamMax=[]  KtParamMin=[]  KtParamMax=[]  POutMin=[]  POutMax=[]  IOutMin=[]  IOutMax=[]  DOutMin=[]  DOutMax=[]  NOutMin=[]  NOutMax=[]  bOutMin=[]  bOutMax=[]  cOutMin=[]  cOutMax=[]  KbOutMin=[]  KbOutMax=[]  KtOutMin=[]  KtOutMax=[]  IntegratorOutMin=[]  IntegratorOutMax=[]  FilterOutMin=[]  FilterOutMax=[]  SumOutMin=[]  SumOutMax=[]  Sum1OutMin=[]  Sum1OutMax=[]  Sum2OutMin=[]  Sum2OutMax=[]  Sum3OutMin=[]  Sum3OutMax=[]  SumI1OutMin=[]  SumI1OutMax=[]  SumI2OutMin=[]  SumI2OutMax=[]  SumI3OutMin=[]  SumI3OutMax=[]  SumDOutMin=[]  SumDOutMax=[]  SaturationOutMin=[]  SaturationOutMax=[]  IntegratorContinuousStateAttributes=''  IntegratorStateMustResolveToSignalObject=off  IntegratorRTWStateStorageClass=Auto  FilterContinuousStateAttributes=''  FilterStateMustResolveToSignalObject=off  FilterRTWStateStorageClass=Auto  DifferentiatorICPrevScaledInput=0  DifferentiatorOutMin=[]  DifferentiatorOutMax=[]  FilterDiffOutCoefMin=[]  FilterDiffOutCoefMax=[]  SumDenOutMin=[]  SumDenOutMax=[]  SumNumOutMin=[]  SumNumOutMax=[]  ReciprocalOutMin=[]  ReciprocalOutMax=[]  DivideOutMin=[]  DivideOutMax=[]  TunerSelectOption=Transfer Function Based (PID Tuner App)
  cfblk15 : DiscreteFir
  cfblk{7,17..19} (4 alike) : Delay
  cfblk3 : DiscreteFir
  cfblk4 : Subsystem  TreatAsAtomicUnit=on
  cfblk5 : Subsystem  TreatAsAtomicUnit=on
  cfblk6 : Subsystem  TreatAsAtomicUnit=on
  cfblk8 : DiscreteZeroPole  Poles=[0 0.5]  Gain=1  SampleTime=-1
  cfblk9 : simulink/Discrete/Transfer Fcn Real Zero  ZeroZ=0.75  ICPrevInput=0.0  DoSatur=off
      settings: SourceProductName=Simulink  SourceProductBaseCode=SL
  cyemi_{537..554} (18 alike) : DataTypeConversion  OutDataTypeStr=double
  emi_1003 : Subsystem  TreatAsAtomicUnit=on
  emi_{261,412,1005,1068,1097} (5 alike) : If  IfExpression=Inf <= u1
  emi_{262,413,1006,1069,1098} (5 alike) : DataTypeConversion  OutDataTypeStr=double
  emi_1066 : Subsystem  TreatAsAtomicUnit=on
  emi_1095 : Subsystem  TreatAsAtomicUnit=on
  emi_259 : Subsystem  TreatAsAtomicUnit=on
  emi_410 : Subsystem  TreatAsAtomicUnit=on
  cfblk2 : Outport
  cfblk16 : Outport  Port=2
  wires:
  cfblk10/1 -> cfblk2/1, cyemi_544/1
  cfblk9/1 -> cfblk16/1
  cyemi_537/1 -> cfblk10/1
  cfblk8/1 -> cyemi_537/1
  cyemi_538/1 -> cfblk11/1
  cfblk14/1 -> cyemi_538/1
  cfblk11/1 -> cyemi_540/1
  cyemi_541/1 -> cfblk14/1
  cfblk18/1 -> cyemi_541/1
  cyemi_542/1 -> cfblk14/2
  cfblk7/1 -> cyemi_542/1, emi_262/1
  cyemi_543/1 -> cfblk15/1
  cyemi_544/1 -> cfblk17/1
  cyemi_545/1 -> cfblk18/1
  cfblk15/1 -> cyemi_545/1
  cyemi_546/1 -> cfblk19/1
  cyemi_547/1 -> cfblk3/1
  cfblk17/1 -> cyemi_547/1, emi_1006/1
  cfblk3/1 -> cyemi_548/1, emi_1069/1, emi_1098/1
  cfblk19/1 -> cyemi_551/1, emi_413/1
  cyemi_552/1 -> cfblk7/1
  cyemi_553/1 -> cfblk8/1
  cyemi_554/1 -> cfblk9/1
  cfblk1/1 -> cyemi_554/1
  cyemi_551/1 -> cfblk6/1(emi_257)
  cfblk6/1(emi_258) -> cyemi_550/1, cyemi_539/1
  emi_261/1 -> cfblk6/Action
  emi_261/2 -> emi_259/Action
  emi_262/1 -> emi_261/1
  cyemi_539/1 -> cfblk12/1(emi_408)
  cfblk12/1(emi_409) -> cyemi_552/1
  emi_412/1 -> cfblk12/Action
  emi_412/2 -> emi_410/Action
  emi_413/1 -> emi_412/1
  cyemi_548/1 -> cfblk4/1(emi_1001)
  cfblk4/1(emi_1002) -> cyemi_549/1
  emi_1005/1 -> cfblk4/Action
  emi_1005/2 -> emi_1003/Action
  emi_1006/1 -> emi_1005/1
  cyemi_540/1 -> cfblk13/1(emi_1064)
  cfblk13/1(emi_1065) -> cyemi_546/1, cyemi_543/1
  emi_1068/1 -> cfblk13/Action
  emi_1068/2 -> emi_1066/Action
  emi_1069/1 -> emi_1068/1
  cyemi_549/1 -> cfblk5/1(emi_1092)
  cyemi_550/1 -> cfblk5/2(emi_1093)
  cfblk5/1(emi_1094) -> cyemi_553/1
  emi_1097/1 -> cfblk5/Action
  emi_1097/2 -> emi_1095/Action
  emi_1098/1 -> emi_1097/1

== system sampleModel7293_pp_1_1/cfblk184/cfblk17 ==
  cfblk1 : Inport
  Action Port : ActionPort  ActionType=else
  cfblk10 : simulink/Continuous/PID Controller (2DOF)  Controller=PID  TimeDomain=Discrete-time  SampleTime=-1  IntegratorMethod=Forward Euler  FilterMethod=Forward Euler  Form=Parallel  UseFilter=on  ControllerParametersSource=internal  P=1  I=1  D=0  N=100  b=1  c=1  InitialConditionSource=internal  InitialConditionForIntegrator=0  InitialConditionForFilter=0  ExternalReset=none  LimitOutput=off  UpperSaturationLimit=inf  LowerSaturationLimit=-inf  LinearizeAsGain=off  AntiWindupMode=none  Kb=1  TrackingMode=off  Kt=1  PParamMin=[]  PParamMax=[]  IParamMin=[]  IParamMax=[]  DParamMin=[]  DParamMax=[]  NParamMin=[]  NParamMax=[]  bParamMin=[]  bParamMax=[]  cParamMin=[]  cParamMax=[]  KbParamMin=[]  KbParamMax=[]  KtParamMin=[]  KtParamMax=[]  POutMin=[]  POutMax=[]  IOutMin=[]  IOutMax=[]  DOutMin=[]  DOutMax=[]  NOutMin=[]  NOutMax=[]  bOutMin=[]  bOutMax=[]  cOutMin=[]  cOutMax=[]  KbOutMin=[]  KbOutMax=[]  KtOutMin=[]  KtOutMax=[]  IntegratorOutMin=[]  IntegratorOutMax=[]  FilterOutMin=[]  FilterOutMax=[]  SumOutMin=[]  SumOutMax=[]  Sum1OutMin=[]  Sum1OutMax=[]  Sum2OutMin=[]  Sum2OutMax=[]  Sum3OutMin=[]  Sum3OutMax=[]  SumI1OutMin=[]  SumI1OutMax=[]  SumI2OutMin=[]  SumI2OutMax=[]  SumI3OutMin=[]  SumI3OutMax=[]  SumDOutMin=[]  SumDOutMax=[]  SaturationOutMin=[]  SaturationOutMax=[]  IntegratorContinuousStateAttributes=''  IntegratorStateMustResolveToSignalObject=off  IntegratorRTWStateStorageClass=Auto  FilterContinuousStateAttributes=''  FilterStateMustResolveToSignalObject=off  FilterRTWStateStorageClass=Auto  DifferentiatorICPrevScaledInput=0  DifferentiatorOutMin=[]  DifferentiatorOutMax=[]  FilterDiffOutCoefMin=[]  FilterDiffOutCoefMax=[]  SumDenOutMin=[]  SumDenOutMax=[]  SumNumOutMin=[]  SumNumOutMax=[]  ReciprocalOutMin=[]  ReciprocalOutMax=[]  DivideOutMin=[]  DivideOutMax=[]  TunerSelectOption=Transfer Function Based (PID Tuner App)
  cfblk11 : UnitDelay  SampleTime=-1
  cfblk12 : simulink/Continuous/PID Controller (2DOF)  Controller=PID  TimeDomain=Discrete-time  SampleTime=-1  IntegratorMethod=Forward Euler  FilterMethod=Forward Euler  Form=Parallel  UseFilter=on  ControllerParametersSource=internal  P=1  I=1  D=0  N=100  b=1  c=1  InitialConditionSource=internal  InitialConditionForIntegrator=0  InitialConditionForFilter=0  ExternalReset=none  LimitOutput=off  UpperSaturationLimit=inf  LowerSaturationLimit=-inf  LinearizeAsGain=off  AntiWindupMode=none  Kb=1  TrackingMode=off  Kt=1  PParamMin=[]  PParamMax=[]  IParamMin=[]  IParamMax=[]  DParamMin=[]  DParamMax=[]  NParamMin=[]  NParamMax=[]  bParamMin=[]  bParamMax=[]  cParamMin=[]  cParamMax=[]  KbParamMin=[]  KbParamMax=[]  KtParamMin=[]  KtParamMax=[]  POutMin=[]  POutMax=[]  IOutMin=[]  IOutMax=[]  DOutMin=[]  DOutMax=[]  NOutMin=[]  NOutMax=[]  bOutMin=[]  bOutMax=[]  cOutMin=[]  cOutMax=[]  KbOutMin=[]  KbOutMax=[]  KtOutMin=[]  KtOutMax=[]  IntegratorOutMin=[]  IntegratorOutMax=[]  FilterOutMin=[]  FilterOutMax=[]  SumOutMin=[]  SumOutMax=[]  Sum1OutMin=[]  Sum1OutMax=[]  Sum2OutMin=[]  Sum2OutMax=[]  Sum3OutMin=[]  Sum3OutMax=[]  SumI1OutMin=[]  SumI1OutMax=[]  SumI2OutMin=[]  SumI2OutMax=[]  SumI3OutMin=[]  SumI3OutMax=[]  SumDOutMin=[]  SumDOutMax=[]  SaturationOutMin=[]  SaturationOutMax=[]  IntegratorContinuousStateAttributes=''  IntegratorStateMustResolveToSignalObject=off  IntegratorRTWStateStorageClass=Auto  FilterContinuousStateAttributes=''  FilterStateMustResolveToSignalObject=off  FilterRTWStateStorageClass=Auto  DifferentiatorICPrevScaledInput=0  DifferentiatorOutMin=[]  DifferentiatorOutMax=[]  FilterDiffOutCoefMin=[]  FilterDiffOutCoefMax=[]  SumDenOutMin=[]  SumDenOutMax=[]  SumNumOutMin=[]  SumNumOutMax=[]  ReciprocalOutMin=[]  ReciprocalOutMax=[]  DivideOutMin=[]  DivideOutMax=[]  TunerSelectOption=Transfer Function Based (PID Tuner App)
  cfblk13 : DiscreteFir
  cfblk14 : Subsystem  TreatAsAtomicUnit=on
  cfblk16 : Delay
  cfblk17 : Delay
  cfblk3 : simulink/Discrete/Transfer Fcn Real Zero  ZeroZ=0.75  ICPrevInput=0.0  DoSatur=off
      settings: SourceProductName=Simulink  SourceProductBaseCode=SL
  cfblk4 : simulink/Discrete/Difference  ICPrevInput=0.0  OutMin=[]  OutMax=[]  OutDataTypeStr=double  OutputDataTypeScalingMode=double  OutDataType=fixdt(1, 16)  OutScaling=2^-10  DoSatur=off
  cfblk5 : UnitDelay  SampleTime=-1
  cfblk6 : Delay
  cfblk7 : DiscreteStateSpace  SampleTime=-1
  cfblk8 : Subsystem  TreatAsAtomicUnit=on
  cfblk9 : Subsystem  TreatAsAtomicUnit=on
  cyemi_{556..571} (16 alike) : DataTypeConversion  OutDataTypeStr=double
  emi_1204 : Subsystem  TreatAsAtomicUnit=on
  emi_1206 : If  IfExpression=Inf <= u1
  emi_1207 : DataTypeConversion  OutDataTypeStr=double
  emi_1922 : Subsystem  TreatAsAtomicUnit=on
  emi_1924 : If  IfExpression=Inf <= u1
  emi_1925 : DataTypeConversion  OutDataTypeStr=double
  emi_940 : Subsystem  TreatAsAtomicUnit=on
  emi_942 : If  IfExpression=Inf <= u1
  emi_943 : DataTypeConversion  OutDataTypeStr=double
  cfblk2 : Outport
  cfblk15 : Outport  Port=2
  wires:
  cfblk4/1 -> cfblk15/1, cyemi_570/1
  cfblk7/1 -> cyemi_557/1, cyemi_560/1, emi_1207/1
  cfblk13/1 -> cyemi_556/1, cyemi_566/1
  cfblk11/1 -> cfblk2/1
  cyemi_556/1 -> cfblk10/1
  cyemi_557/1 -> cfblk10/2
  cyemi_558/1 -> cfblk11/1
  cfblk10/1 -> cyemi_558/1
  cyemi_559/1 -> cfblk12/1
  cfblk16/1 -> cyemi_559/1
  cyemi_560/1 -> cfblk12/2
  cyemi_561/1 -> cfblk13/1
  cfblk12/1 -> cyemi_562/1
  cyemi_563/1 -> cfblk16/1
  cyemi_564/1 -> cfblk17/1
  cfblk6/1 -> cyemi_564/1
  cyemi_565/1 -> cfblk3/1
  cfblk17/1 -> cyemi_565/1
  cyemi_566/1 -> cfblk4/1
  cyemi_567/1 -> cfblk5/1
  cfblk1/1 -> cyemi_567/1
  cyemi_568/1 -> cfblk6/1
  cyemi_569/1 -> cfblk7/1
  cfblk5/1 -> cyemi_569/1, emi_1925/1
  cfblk3/1 -> cyemi_571/1
  cyemi_570/1 -> cfblk8/1(emi_938)
  cfblk8/1(emi_939) -> cyemi_563/1
  emi_942/1 -> cfblk8/Action
  emi_942/2 -> emi_940/Action
  emi_943/1 -> emi_942/1
  cyemi_571/1 -> cfblk9/1(emi_1202)
  cfblk9/1(emi_1203) -> emi_943/1, cyemi_568/1
  emi_1206/1 -> cfblk9/Action
  emi_1206/2 -> emi_1204/Action
  emi_1207/1 -> emi_1206/1
  cyemi_562/1 -> cfblk14/1(emi_1920)
  cfblk14/1(emi_1921) -> cyemi_561/1
  emi_1924/1 -> cfblk14/Action
  emi_1924/2 -> emi_1922/Action
  emi_1925/1 -> emi_1924/1

== system sampleModel7293_pp_1_1/cfblk184/cfblk8 ==
  emi_1749 : Inport
  Action Port : ActionPort  ActionType=then
  cfblk8 : UnitDelay  SampleTime=-1
  emi_1750 : Outport
  wires:
  emi_1749/1 -> cfblk8/1
  cfblk8/1 -> emi_1750/1

== system sampleModel7293_pp_1_1/cfblk184/emi_1751 ==
  Action Port : ActionPort  ActionType=else
  emi_1752 : Assertion

== system sampleModel7293_pp_1_1/cfblk184/emi_856 ==
  Action Port : ActionPort  ActionType=else
  emi_857 : Assertion

== system sampleModel7293_pp_1_1/cfblk185/cfblk18 ==
  cfblk1 : Inport
  cfblk11 : Inport  Port=2
  Action Port : ActionPort  ActionType=then
  cfblk10 : DiscreteZeroPole  Poles=[0 0.5]  Gain=1  SampleTime=-1
  cfblk13 : Delay
  cfblk14 : Delay
  cfblk3 : DiscreteStateSpace  SampleTime=-1
  cfblk4 : Subsystem  TreatAsAtomicUnit=on
  cfblk5 : Subsystem  TreatAsAtomicUnit=on
  cfblk6 : DiscreteZeroPole  Poles=[0 0.5]  Gain=1  SampleTime=-1
  cfblk7 : simulink/Discrete/Difference  ICPrevInput=0.0  OutMin=[]  OutMax=[]  OutDataTypeStr=double  OutputDataTypeScalingMode=double  OutDataType=fixdt(1, 16)  OutScaling=2^-10  DoSatur=off
  cfblk8 : simulink/Discrete/Difference  ICPrevInput=0.0  OutMin=[]  OutMax=[]  OutDataTypeStr=double  OutputDataTypeScalingMode=double  OutDataType=fixdt(1, 16)  OutScaling=2^-10  DoSatur=off
  cfblk9 : DiscreteFilter
  cyemi_{596..606} (11 alike) : DataTypeConversion  OutDataTypeStr=double
  emi_1831 : Subsystem  TreatAsAtomicUnit=on
  emi_1833 : If  IfExpression=0 <= u1
  emi_1834 : DataTypeConversion  OutDataTypeStr=double
  emi_655 : Subsystem  TreatAsAtomicUnit=on
  emi_657 : If  IfExpression=0 <= u1
  emi_658 : DataTypeConversion  OutDataTypeStr=double
  cfblk2 : Outport
  cfblk12 : Outport  Port=2
  wires:
  cfblk8/1 -> cfblk12/1
  cfblk6/1 -> cfblk2/1, cyemi_606/1, emi_658/1
  cyemi_596/1 -> cfblk10/1
  cfblk3/1 -> cyemi_596/1
  cyemi_597/1 -> cfblk13/1
  cfblk7/1 -> cyemi_597/1
  cyemi_598/1 -> cfblk14/1
  cfblk10/1 -> cyemi_598/1
  cyemi_599/1 -> cfblk3/1
  cfblk14/1 -> cyemi_599/1
  cfblk1/1 -> cyemi_600/1
  cfblk13/1 -> cyemi_601/1
  cfblk9/1 -> cyemi_602/1, emi_1834/1
  cyemi_603/1 -> cfblk6/1
  cfblk11/1 -> cyemi_603/1
  cyemi_604/1 -> cfblk7/1
  cyemi_605/1 -> cfblk8/1
  cyemi_606/1 -> cfblk9/1
  cyemi_602/1 -> cfblk5/1(emi_653)
  cfblk5/1(emi_654) -> cyemi_605/1
  emi_657/1 -> cfblk5/Action
  emi_657/2 -> emi_655/Action
  emi_658/1 -> emi_657/1
  cyemi_600/1 -> cfblk4/1(emi_1828)
  cyemi_601/1 -> cfblk4/2(emi_1829)
  cfblk4/1(emi_1830) -> cyemi_604/1
  emi_1833/1 -> cfblk4/Action
  emi_1833/2 -> emi_1831/Action
  emi_1834/1 -> emi_1833/1
